simulink model "Simulink_ADC"  (R2016a)
settings: Solver=ode1  StartTime=0.0  StopTime=50  FixedStep=1e-6  RelTol=1e-3
libraries: commdigbbndpm3 x2, commchan3 x1, commsink2 x1, commrandsrc3 x1, dspquant2 x1
settings Model: Creator=LENOVO  LastModifiedBy=LENOVO

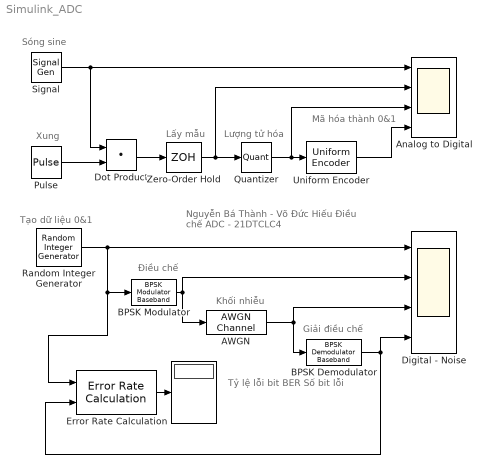
== system Simulink_ADC ==
  note: Điều chế
  note: Giải điều chế
  note: Tỷ lệ lỗi bit
      | BER
      | Số bit lỗi
  note: Xung
  note: Sóng sine
  note: Tạo dữ liệu 0&1
  note: Khối nhiễu
  note: Mã hóa
      | thành 0&1
  note: Lượng tử hóa
  note: Lấy mẫu
  note: Nguyễn Bá Thành - Võ Đức Hiếu
      | Điều chế ADC - 21DTCLC4
  " " : Display
  "AWGN " : commchan3/AWGN Channel  InputProcessing=Columns as channels (frame based)  seed=67  noiseMode="Signal to noise ratio  (Es/No)"  EbNodB=1  EsNodB=1e-6  SNRdB=10  bitsPerSym=1  Ps=1  Tsym=1  variance=1000
  Analog to Digital : Scope  NumInputPorts=4
  "BPSK Demodulator " : commdigbbndpm3/BPSK Demodulator Baseband  DecType=Hard decision  VarSource=Dialog  Variance=1  Ph=0  outDtype=Inherit via internal rule  derotateFactorWordLen=16  derotateFactorDataTypeStr=Inherit: Same word length as input  derotateFactorLastDataTypeStr=Inherit: Same word length as input
  "BPSK Modulator " : commdigbbndpm3/BPSK Modulator Baseband  Ph=0  outDtype=double  outWordLen=16  outUDDataType=sfix(16)  outFracLenMode=Best precision  outFracLen=15  outDataTypeStr=double  outLastDataTypeStr=double
  Digital - Noise : Scope  NumInputPorts=4
  Dot Product : DotProduct  InputSameDT=on  OutDataTypeStr=Inherit: Inherit via internal rule
  Error Rate Calculation : commsink2/Error Rate Calculation  N=0  st_delay=0  cp_mode=Entire frame  subframe=[]  PMode=Port  WsName=ErrorVec  RsMode2=off  stop=on  numErr=100  maxBits=1e5
  "Pulse " : DiscretePulseGenerator  PulseType=Time based  Amplitude=0.75  Period=1  PulseWidth=60  SampleTime=1e-6
  Quantizer : Quantizer  QuantizationInterval=0.66
  Random Integer Generator : commrandsrc3/Random Integer Generator  SetSize=2  SeedSource=Auto  Seed=0  SampleTime=1  SamplesPerFrame=1  OutputDataType=double  SimulateUsing=Interpreted execution
  "Signal " : SignalGenerator  Amplitude=0.75  Frequency=0.035
  Uniform Encoder : dspquant2/Uniform Encoder  peak=1  bits=2  otype=Unsigned integer
  Zero-Order Hold : ZeroOrderHold  SampleTime=1e-6
  wires:
  "Signal "/1 -> Dot Product/1, Analog to Digital/1
  "Pulse "/1 -> Dot Product/2
  Dot Product/1 -> Zero-Order Hold/1
  Quantizer/1 -> Analog to Digital/3, Uniform Encoder/1
  Error Rate Calculation/1 -> " "/1
  "BPSK Modulator "/1 -> "AWGN "/1, Digital - Noise/2
  "AWGN "/1 -> "BPSK Demodulator "/1, Digital - Noise/3
  "BPSK Demodulator "/1 -> Digital - Noise/4, Error Rate Calculation/2
  Zero-Order Hold/1 -> Quantizer/1, Analog to Digital/2
  Random Integer Generator/1 -> Error Rate Calculation/1, "BPSK Modulator "/1, Digital - Noise/1
  Uniform Encoder/1 -> Analog to Digital/4
